simulink model "Model_turn"  (R2024a)
settings: Solver=VariableStepAuto  StartTime=0.0  StopTime=100  MaxStep=0.1  RelTol=1e-3
values from neighbouring files (symbols this model uses):
  c_SMA = 837.36    [params.m]
  Fmax_SMA = 10    [params.m]
  h_SMA = .3    (= 0.3)    [params.m]
  k_gn = m*g/0.01    (= 9810)    [contact3D_params.m]
  k_gt = m*g/0.1    (= 981)    [contact3D_params.m]
  m = 10    [contact3D_params.m]
  m_SMA = 0.0025    [params.m]
  max_SMA_Energy_J = 150    [params.m]
  mu_slide = 0.8    [contact3D_params.m]
  mu_stick = 0.9    [contact3D_params.m]
  n_segs = 10    [params.m]
  PWM_max = 0.35    [params.m]
  R_SMA = .08    (= 0.08)    [params.m]
  r_SMA2limb = 0.009    [params.m]
  swing_angle = swing_angles(i)    [params.m]
  T_amb = 23    [params.m]
  V_0 = 7    [params.m]
  v_gn_max = 0.03    [contact3D_params.m]
  v_gt_max = 0.03    [contact3D_params.m]
  vLimit = 0.01    [contact3D_params.m]
undefined symbols (not defined in the file or in its folder): Newton, Raphson, X, Y, Z
libraries: sm_lib x225, nesl_utility x185, simulink x24, simulink_extras x6
(part 2 of 16)

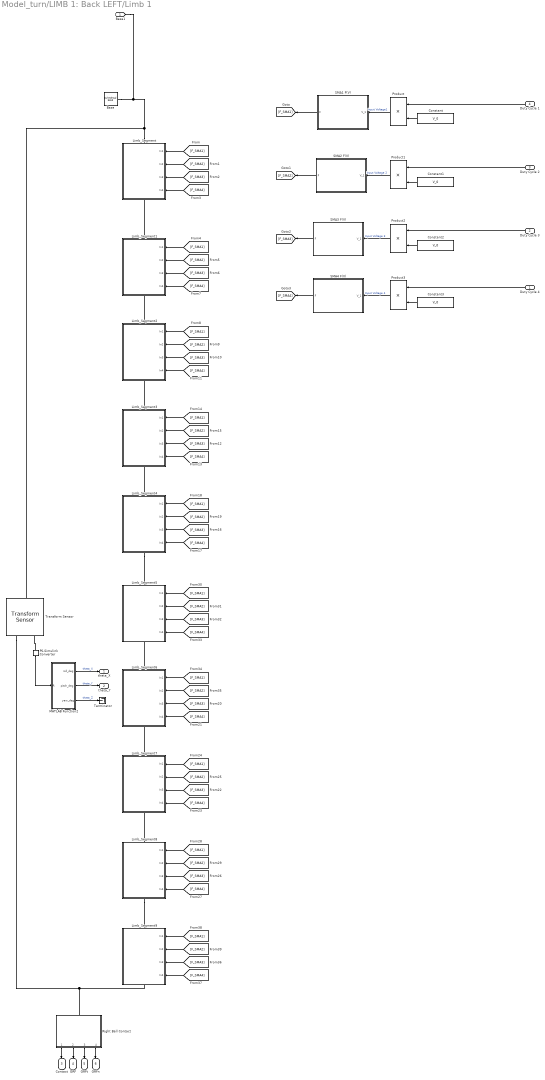
== system Model_turn/LIMB 1: Back LEFT/Limb 1 ==
  Duty Cycle 4 : Inport
  Duty Cycle 3 : Inport  Port=2
  Duty Cycle 2 : Inport  Port=3
  Duty Cycle 1 : Inport  Port=4
  Base : sm_lib/Body Elements/Cylindrical Solid  CylinderRadius=rad_limb  CylinderRadiusUnits=m  CylinderLength=seg_length  CylinderLengthUnits=m  ExportEntireGeometry=off  InertiaType=CalculateFromGeometry  BasedOnType=Density  Density=limb_density  DensityUnits=kg/m^3  Mass=1  MassUnits=kg  CenterOfMass=[0 0 0]  CenterOfMassUnits=m  MomentsOfInertia=[1 1 1]  MomentsOfInertiaUnits=kg*m^2  ProductsOfInertia=[0 0 0]  ProductsOfInertiaUnits=kg*m^2  GraphicType=FromGeometry  MarkerShape=Sphere  MarkerSize=10  GraphicVisPropType=SimpleVisualProperties  GraphicDiffuseColor=[0.5 0.5 0.5]  GraphicOpacity=1  GraphicSpecularColor=[0.5 0.5 0.5 1.0]  GraphicAmbientColor=[0.15 0.15 0.15 1.0]  GraphicEmissiveColor=[0.0 0.0 0.0 1.0]  GraphicShininess=75  DoExposeReferenceFrame=on  SerializedFrames=<Frames/>
  Constant{,1..3} (4 alike) : Constant  Value=V_0
  Limb_Segment : Subsystem
      settings: PortSchema="{\"entries\":[{\"content\":{\"sides\":[{\"content\":{\"connectorIds\":[\"In1\",\"In2\",\"In3\",\"In4\"]},\"type\":\"ConnectorPlacement.EquallySpacedRectSide\",\"uuid\":\"d6f10fa6-a397-4eb1-90c1-ee7478ada294\"},{\"content\":{\"side\":\"RIGHT\"},\"type\":\"ConnectorPlacement.EquallySpacedRectSide\",\"uuid\":\"3f1db35a-8e6d-4ba3-9e2d-f9910440e53b\"},{\"content\":{\"connectorIds\":[\"LConn1\"],\"side\":\"TOP\"},\"type\":\"ConnectorPlacement.EquallySpacedRectSide\",\"uuid\":\"a4104d1f-7883-4f84-b664-87694b536b33\"},{\"content\":{\"connectorIds\":[\"RConn1\"],\"side\":\"BOTTOM\"},\"type\":\"ConnectorPlacement.EquallySpacedRectSide\",\"uuid\":\"6469b369-5782-4c2c-b5b8-85624622bc1d\"}]},\"type\":\"ConnectorPlacement.EquallySpacedConnector\",\"uuid\":\"3cfa1fa9-4e06-4e7e-9a4a-6c954422b5b2\"}],\"packageUris\":[\"http://schema.mathworks.com/mf0/Connector/R2020b\"],\"version\":\"1.0\"}"
  Limb_Segment1 : Subsystem
      settings: PortSchema="{\"entries\":[{\"content\":{\"sides\":[{\"content\":{\"connectorIds\":[\"In1\",\"In2\",\"In3\",\"In4\"]},\"type\":\"ConnectorPlacement.EquallySpacedRectSide\",\"uuid\":\"d6f10fa6-a397-4eb1-90c1-ee7478ada294\"},{\"content\":{\"side\":\"RIGHT\"},\"type\":\"ConnectorPlacement.EquallySpacedRectSide\",\"uuid\":\"3f1db35a-8e6d-4ba3-9e2d-f9910440e53b\"},{\"content\":{\"connectorIds\":[\"LConn1\"],\"side\":\"TOP\"},\"type\":\"ConnectorPlacement.EquallySpacedRectSide\",\"uuid\":\"a4104d1f-7883-4f84-b664-87694b536b33\"},{\"content\":{\"connectorIds\":[\"RConn1\"],\"side\":\"BOTTOM\"},\"type\":\"ConnectorPlacement.EquallySpacedRectSide\",\"uuid\":\"6469b369-5782-4c2c-b5b8-85624622bc1d\"}]},\"type\":\"ConnectorPlacement.EquallySpacedConnector\",\"uuid\":\"3cfa1fa9-4e06-4e7e-9a4a-6c954422b5b2\"}],\"packageUris\":[\"http://schema.mathworks.com/mf0/Connector/R2020b\"],\"version\":\"1.0\"}"
  Limb_Segment2 : Subsystem
      settings: PortSchema="{\"entries\":[{\"content\":{\"sides\":[{\"content\":{\"connectorIds\":[\"In1\",\"In2\",\"In3\",\"In4\"]},\"type\":\"ConnectorPlacement.EquallySpacedRectSide\",\"uuid\":\"d6f10fa6-a397-4eb1-90c1-ee7478ada294\"},{\"content\":{\"side\":\"RIGHT\"},\"type\":\"ConnectorPlacement.EquallySpacedRectSide\",\"uuid\":\"3f1db35a-8e6d-4ba3-9e2d-f9910440e53b\"},{\"content\":{\"connectorIds\":[\"LConn1\"],\"side\":\"TOP\"},\"type\":\"ConnectorPlacement.EquallySpacedRectSide\",\"uuid\":\"a4104d1f-7883-4f84-b664-87694b536b33\"},{\"content\":{\"connectorIds\":[\"RConn1\"],\"side\":\"BOTTOM\"},\"type\":\"ConnectorPlacement.EquallySpacedRectSide\",\"uuid\":\"6469b369-5782-4c2c-b5b8-85624622bc1d\"}]},\"type\":\"ConnectorPlacement.EquallySpacedConnector\",\"uuid\":\"3cfa1fa9-4e06-4e7e-9a4a-6c954422b5b2\"}],\"packageUris\":[\"http://schema.mathworks.com/mf0/Connector/R2020b\"],\"version\":\"1.0\"}"
  Limb_Segment3 : Subsystem
      settings: PortSchema="{\"entries\":[{\"content\":{\"sides\":[{\"content\":{\"connectorIds\":[\"In1\",\"In2\",\"In3\",\"In4\"]},\"type\":\"ConnectorPlacement.EquallySpacedRectSide\",\"uuid\":\"d6f10fa6-a397-4eb1-90c1-ee7478ada294\"},{\"content\":{\"side\":\"RIGHT\"},\"type\":\"ConnectorPlacement.EquallySpacedRectSide\",\"uuid\":\"3f1db35a-8e6d-4ba3-9e2d-f9910440e53b\"},{\"content\":{\"connectorIds\":[\"LConn1\"],\"side\":\"TOP\"},\"type\":\"ConnectorPlacement.EquallySpacedRectSide\",\"uuid\":\"a4104d1f-7883-4f84-b664-87694b536b33\"},{\"content\":{\"connectorIds\":[\"RConn1\"],\"side\":\"BOTTOM\"},\"type\":\"ConnectorPlacement.EquallySpacedRectSide\",\"uuid\":\"6469b369-5782-4c2c-b5b8-85624622bc1d\"}]},\"type\":\"ConnectorPlacement.EquallySpacedConnector\",\"uuid\":\"3cfa1fa9-4e06-4e7e-9a4a-6c954422b5b2\"}],\"packageUris\":[\"http://schema.mathworks.com/mf0/Connector/R2020b\"],\"version\":\"1.0\"}"
  Limb_Segment4 : Subsystem
      settings: PortSchema="{\"entries\":[{\"content\":{\"sides\":[{\"content\":{\"connectorIds\":[\"In1\",\"In2\",\"In3\",\"In4\"]},\"type\":\"ConnectorPlacement.EquallySpacedRectSide\",\"uuid\":\"d6f10fa6-a397-4eb1-90c1-ee7478ada294\"},{\"content\":{\"side\":\"RIGHT\"},\"type\":\"ConnectorPlacement.EquallySpacedRectSide\",\"uuid\":\"3f1db35a-8e6d-4ba3-9e2d-f9910440e53b\"},{\"content\":{\"connectorIds\":[\"LConn1\"],\"side\":\"TOP\"},\"type\":\"ConnectorPlacement.EquallySpacedRectSide\",\"uuid\":\"a4104d1f-7883-4f84-b664-87694b536b33\"},{\"content\":{\"connectorIds\":[\"RConn1\"],\"side\":\"BOTTOM\"},\"type\":\"ConnectorPlacement.EquallySpacedRectSide\",\"uuid\":\"6469b369-5782-4c2c-b5b8-85624622bc1d\"}]},\"type\":\"ConnectorPlacement.EquallySpacedConnector\",\"uuid\":\"3cfa1fa9-4e06-4e7e-9a4a-6c954422b5b2\"}],\"packageUris\":[\"http://schema.mathworks.com/mf0/Connector/R2020b\"],\"version\":\"1.0\"}"
  Limb_Segment5 : Subsystem
      settings: PortSchema="{\"entries\":[{\"content\":{\"sides\":[{\"content\":{\"connectorIds\":[\"In1\",\"In2\",\"In3\",\"In4\"]},\"type\":\"ConnectorPlacement.EquallySpacedRectSide\",\"uuid\":\"d6f10fa6-a397-4eb1-90c1-ee7478ada294\"},{\"content\":{\"side\":\"RIGHT\"},\"type\":\"ConnectorPlacement.EquallySpacedRectSide\",\"uuid\":\"3f1db35a-8e6d-4ba3-9e2d-f9910440e53b\"},{\"content\":{\"connectorIds\":[\"LConn1\"],\"side\":\"TOP\"},\"type\":\"ConnectorPlacement.EquallySpacedRectSide\",\"uuid\":\"a4104d1f-7883-4f84-b664-87694b536b33\"},{\"content\":{\"connectorIds\":[\"RConn1\"],\"side\":\"BOTTOM\"},\"type\":\"ConnectorPlacement.EquallySpacedRectSide\",\"uuid\":\"6469b369-5782-4c2c-b5b8-85624622bc1d\"}]},\"type\":\"ConnectorPlacement.EquallySpacedConnector\",\"uuid\":\"3cfa1fa9-4e06-4e7e-9a4a-6c954422b5b2\"}],\"packageUris\":[\"http://schema.mathworks.com/mf0/Connector/R2020b\"],\"version\":\"1.0\"}"
  Limb_Segment6 : Subsystem
      settings: PortSchema="{\"entries\":[{\"content\":{\"sides\":[{\"content\":{\"connectorIds\":[\"In1\",\"In2\",\"In3\",\"In4\"]},\"type\":\"ConnectorPlacement.EquallySpacedRectSide\",\"uuid\":\"d6f10fa6-a397-4eb1-90c1-ee7478ada294\"},{\"content\":{\"side\":\"RIGHT\"},\"type\":\"ConnectorPlacement.EquallySpacedRectSide\",\"uuid\":\"3f1db35a-8e6d-4ba3-9e2d-f9910440e53b\"},{\"content\":{\"connectorIds\":[\"LConn1\"],\"side\":\"TOP\"},\"type\":\"ConnectorPlacement.EquallySpacedRectSide\",\"uuid\":\"a4104d1f-7883-4f84-b664-87694b536b33\"},{\"content\":{\"connectorIds\":[\"RConn1\"],\"side\":\"BOTTOM\"},\"type\":\"ConnectorPlacement.EquallySpacedRectSide\",\"uuid\":\"6469b369-5782-4c2c-b5b8-85624622bc1d\"}]},\"type\":\"ConnectorPlacement.EquallySpacedConnector\",\"uuid\":\"3cfa1fa9-4e06-4e7e-9a4a-6c954422b5b2\"}],\"packageUris\":[\"http://schema.mathworks.com/mf0/Connector/R2020b\"],\"version\":\"1.0\"}"
  Limb_Segment7 : Subsystem
      settings: PortSchema="{\"entries\":[{\"content\":{\"sides\":[{\"content\":{\"connectorIds\":[\"In1\",\"In2\",\"In3\",\"In4\"]},\"type\":\"ConnectorPlacement.EquallySpacedRectSide\",\"uuid\":\"d6f10fa6-a397-4eb1-90c1-ee7478ada294\"},{\"content\":{\"side\":\"RIGHT\"},\"type\":\"ConnectorPlacement.EquallySpacedRectSide\",\"uuid\":\"3f1db35a-8e6d-4ba3-9e2d-f9910440e53b\"},{\"content\":{\"connectorIds\":[\"LConn1\"],\"side\":\"TOP\"},\"type\":\"ConnectorPlacement.EquallySpacedRectSide\",\"uuid\":\"a4104d1f-7883-4f84-b664-87694b536b33\"},{\"content\":{\"connectorIds\":[\"RConn1\"],\"side\":\"BOTTOM\"},\"type\":\"ConnectorPlacement.EquallySpacedRectSide\",\"uuid\":\"6469b369-5782-4c2c-b5b8-85624622bc1d\"}]},\"type\":\"ConnectorPlacement.EquallySpacedConnector\",\"uuid\":\"3cfa1fa9-4e06-4e7e-9a4a-6c954422b5b2\"}],\"packageUris\":[\"http://schema.mathworks.com/mf0/Connector/R2020b\"],\"version\":\"1.0\"}"
  Limb_Segment8 : Subsystem
      settings: PortSchema="{\"entries\":[{\"content\":{\"sides\":[{\"content\":{\"connectorIds\":[\"In1\",\"In2\",\"In3\",\"In4\"]},\"type\":\"ConnectorPlacement.EquallySpacedRectSide\",\"uuid\":\"d6f10fa6-a397-4eb1-90c1-ee7478ada294\"},{\"content\":{\"side\":\"RIGHT\"},\"type\":\"ConnectorPlacement.EquallySpacedRectSide\",\"uuid\":\"3f1db35a-8e6d-4ba3-9e2d-f9910440e53b\"},{\"content\":{\"connectorIds\":[\"LConn1\"],\"side\":\"TOP\"},\"type\":\"ConnectorPlacement.EquallySpacedRectSide\",\"uuid\":\"a4104d1f-7883-4f84-b664-87694b536b33\"},{\"content\":{\"connectorIds\":[\"RConn1\"],\"side\":\"BOTTOM\"},\"type\":\"ConnectorPlacement.EquallySpacedRectSide\",\"uuid\":\"6469b369-5782-4c2c-b5b8-85624622bc1d\"}]},\"type\":\"ConnectorPlacement.EquallySpacedConnector\",\"uuid\":\"3cfa1fa9-4e06-4e7e-9a4a-6c954422b5b2\"}],\"packageUris\":[\"http://schema.mathworks.com/mf0/Connector/R2020b\"],\"version\":\"1.0\"}"
  Limb_Segment9 : Subsystem
      settings: PortSchema="{\"entries\":[{\"content\":{\"sides\":[{\"content\":{\"connectorIds\":[\"In1\",\"In2\",\"In3\",\"In4\"]},\"type\":\"ConnectorPlacement.EquallySpacedRectSide\",\"uuid\":\"d6f10fa6-a397-4eb1-90c1-ee7478ada294\"},{\"content\":{\"side\":\"RIGHT\"},\"type\":\"ConnectorPlacement.EquallySpacedRectSide\",\"uuid\":\"3f1db35a-8e6d-4ba3-9e2d-f9910440e53b\"},{\"content\":{\"connectorIds\":[\"LConn1\"],\"side\":\"TOP\"},\"type\":\"ConnectorPlacement.EquallySpacedRectSide\",\"uuid\":\"a4104d1f-7883-4f84-b664-87694b536b33\"},{\"content\":{\"connectorIds\":[\"RConn1\"],\"side\":\"BOTTOM\"},\"type\":\"ConnectorPlacement.EquallySpacedRectSide\",\"uuid\":\"6469b369-5782-4c2c-b5b8-85624622bc1d\"}]},\"type\":\"ConnectorPlacement.EquallySpacedConnector\",\"uuid\":\"3cfa1fa9-4e06-4e7e-9a4a-6c954422b5b2\"}],\"packageUris\":[\"http://schema.mathworks.com/mf0/Connector/R2020b\"],\"version\":\"1.0\"}"
  MATLAB Function2 : MATLAB Function  TreatAsAtomicUnit=on
  PS-Simulink Converter : nesl_utility/PS-Simulink Converter  PhysicalDomain=network_engine_domain  SubClassName=ps_output  LeftPortType=input  RightPortType=output  PseudoPeriodic=off  Frequencies=[]  VectorFormat=inherit  Unit=inherit  AffineConversion=off
  Product{,1..3} (4 alike) : Product
  Right Ball Contact : Subsystem
  SMA1 F(V) : Subsystem
  SMA2 F(V) : Subsystem
  SMA3 F(V) : Subsystem
  SMA4 F(V) : Subsystem
  Terminator : Terminator
  Transform Sensor : sm_lib/Frames and Transforms/Transform Sensor  MeasurementFrame=Base  RotationSequence=XYZ  SenseAngle=off  SenseAxis=off  SenseQ=off  SenseR=on  SenseRotationSequence=off  SenseOmegaX=off  SenseOmegaY=off  SenseOmegaZ=off  SenseOmega=off  SenseQDot=off  SenseRDot=off  SenseRotationSequenceDot=off  SenseAlphaX=off  SenseAlphaY=off  SenseAlphaZ=off  SenseAlpha=off  SenseQDDot=off  SenseRDDot=off  SenseX=off  SenseY=off  SenseZ=off  SenseXYZ=off  SenseRad=off  SenseAzim=off  SenseDist=off  SenseInc=off  SenseXDot=off  SenseYDot=off  SenseZDot=off  SenseXYZDot=off  SenseRadDot=off  SenseAzimDot=off  SenseDistDot=off  SenseIncDot=off  SenseXDDot=off  SenseYDDot=off  SenseZDDot=off  SenseXYZDDot=off  SenseRadDDot=off  SenseAzimDDot=off  SenseDistDDot=off  SenseIncDDot=off
  Base1 : PMIOPort  Side=Left
  theta_X : Outport
  theta_Y : Outport  Port=2
  "Contact " : Outport  Port=3
  GRF : Outport  Port=4
  GRFt : Outport  Port=5
  GRFn : Outport  Port=6
  wires:
  Duty Cycle 1/1 -> Product/1
  MATLAB Function2/1(roll_deg) -> theta_X/1  "theta_X"
  MATLAB Function2/2(pitch_deg) -> theta_Y/1  "theta_Y"
  Duty Cycle 2/1 -> Product1/1
  Duty Cycle 3/1 -> Product2/1
  Product1/1 -> SMA2 F(V)/1(V_1)  "Input Voltage 2"
  MATLAB Function2/3(yaw_deg) -> Terminator/1  "theta_Z"
  Product/1 -> SMA1 F(V)/1(V_1)  "Input Voltage1"
  Constant3/1 -> Product3/2
  [F_SMA2] -> Limb_Segment5/2(In2)
  [F_SMA4] -> Limb_Segment7/4(In4)
  [F_SMA4] -> Limb_Segment/4(In4)
  [F_SMA4] -> Limb_Segment2/4(In4)
  [F_SMA1] -> Limb_Segment7/1(In1)
  [F_SMA3] -> Limb_Segment6/3(In3)
  SMA4 F(V)/1(F) -> [F_SMA4]
  [F_SMA1] -> Limb_Segment9/1(In1)
  [F_SMA4] -> Limb_Segment9/4(In4)
  Constant1/1 -> Product1/2
  [F_SMA3] -> Limb_Segment3/3(In3)
  [F_SMA2] -> Limb_Segment6/2(In2)
  Product3/1 -> SMA4 F(V)/1(V_1)  "Input Voltage 4"
  [F_SMA1] -> Limb_Segment/1(In1)
  PS-Simulink Converter/1 -> MATLAB Function2/1(R)
  [F_SMA4] -> Limb_Segment6/4(In4)
  [F_SMA3] -> Limb_Segment8/3(In3)
  [F_SMA1] -> Limb_Segment8/1(In1)
  [F_SMA1] -> Limb_Segment3/1(In1)
  Duty Cycle 4/1 -> Product3/1
  [F_SMA1] -> Limb_Segment5/1(In1)
  [F_SMA1] -> Limb_Segment4/1(In1)
  [F_SMA2] -> Limb_Segment7/2(In2)
  [F_SMA2] -> Limb_Segment2/2(In2)
  SMA2 F(V)/1(F) -> [F_SMA2]
  Product2/1 -> SMA3 F(V)/1(V_1)  "Input Voltage 3"
  [F_SMA3] -> Limb_Segment9/3(In3)
  [F_SMA2] -> Limb_Segment1/2(In2)
  [F_SMA1] -> Limb_Segment2/1(In1)
  [F_SMA3] -> Limb_Segment4/3(In3)
  [F_SMA2] -> Limb_Segment/2(In2)
  [F_SMA3] -> Limb_Segment/3(In3)
  [F_SMA4] -> Limb_Segment3/4(In4)
  [F_SMA4] -> Limb_Segment1/4(In4)
  [F_SMA4] -> Limb_Segment5/4(In4)
  [F_SMA4] -> Limb_Segment4/4(In4)
  Constant/1 -> Product/2
  [F_SMA3] -> Limb_Segment7/3(In3)
  [F_SMA3] -> Limb_Segment5/3(In3)
  [F_SMA4] -> Limb_Segment8/4(In4)
  SMA1 F(V)/1(F) -> [F_SMA1]
  [F_SMA1] -> Limb_Segment6/1(In1)
  Constant2/1 -> Product2/2
  [F_SMA2] -> Limb_Segment9/2(In2)
  [F_SMA3] -> Limb_Segment1/3(In3)
  SMA3 F(V)/1(F) -> [F_SMA3]
  [F_SMA3] -> Limb_Segment2/3(In3)
  [F_SMA2] -> Limb_Segment8/2(In2)
  [F_SMA1] -> Limb_Segment1/1(In1)
  [F_SMA2] -> Limb_Segment3/2(In2)
  [F_SMA2] -> Limb_Segment4/2(In2)
  Right Ball Contact/2(GRF [N N N]) -> GRF/1
  Right Ball Contact/4(GRFn [N N N]) -> GRFn/1
  Right Ball Contact/1(RBallContact [bool]) -> "Contact "/1
  Right Ball Contact/3(GRFt [N N N]) -> GRFt/1
  connections:
  PS-Simulink Converter/LConn1 -- Transform Sensor/RConn2
  Limb_Segment1/LConn1 -- Limb_Segment/RConn1
  Limb_Segment4/RConn1 -- Limb_Segment5/LConn1
  Limb_Segment7/LConn1 -- Limb_Segment6/RConn1
  Transform Sensor/RConn1 -- Right Ball Contact/LConn1 -- Limb_Segment9/RConn1
  Limb_Segment8/LConn1 -- Limb_Segment7/RConn1
  Limb_Segment6/LConn1 -- Limb_Segment5/RConn1
  Limb_Segment4/LConn1 -- Limb_Segment3/RConn1
  Limb_Segment3/LConn1 -- Limb_Segment2/RConn1
  Limb_Segment8/RConn1 -- Limb_Segment9/LConn1
  Limb_Segment2/LConn1 -- Limb_Segment1/RConn1
  Limb_Segment/LConn1 -- Base/RConn1 -- Base1/RConn1 -- Transform Sensor/LConn1

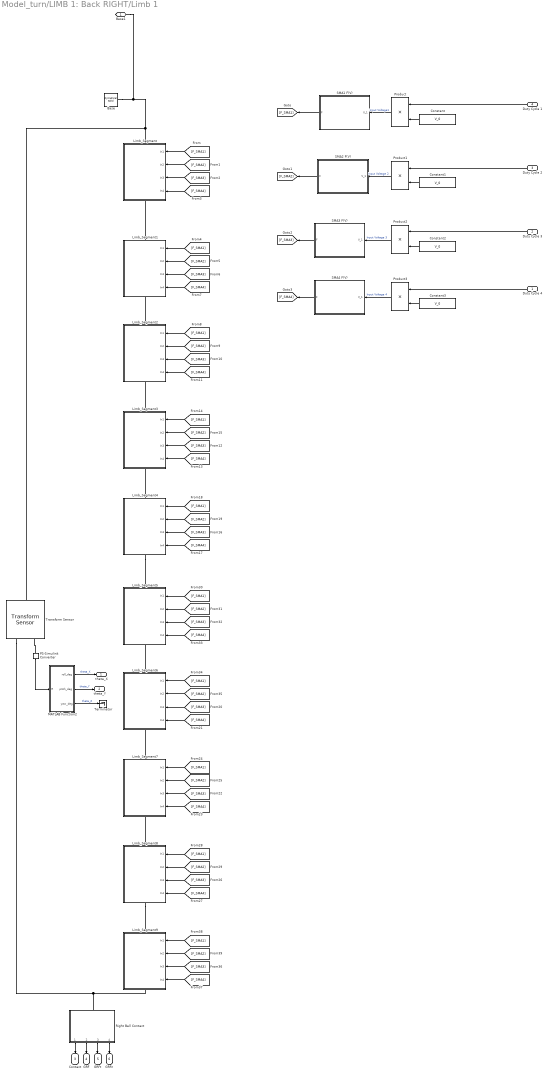
== system Model_turn/LIMB 1: Back RIGHT/Limb 1 ==
  Duty Cycle 4 : Inport
  Duty Cycle 3 : Inport  Port=2
  Duty Cycle 2 : Inport  Port=3
  Duty Cycle 1 : Inport  Port=4
  Base : sm_lib/Body Elements/Cylindrical Solid  CylinderRadius=rad_limb  CylinderRadiusUnits=m  CylinderLength=seg_length  CylinderLengthUnits=m  ExportEntireGeometry=off  InertiaType=CalculateFromGeometry  BasedOnType=Density  Density=limb_density  DensityUnits=kg/m^3  Mass=1  MassUnits=kg  CenterOfMass=[0 0 0]  CenterOfMassUnits=m  MomentsOfInertia=[1 1 1]  MomentsOfInertiaUnits=kg*m^2  ProductsOfInertia=[0 0 0]  ProductsOfInertiaUnits=kg*m^2  GraphicType=FromGeometry  MarkerShape=Sphere  MarkerSize=10  GraphicVisPropType=SimpleVisualProperties  GraphicDiffuseColor=[0.5 0.5 0.5]  GraphicOpacity=1  GraphicSpecularColor=[0.5 0.5 0.5 1.0]  GraphicAmbientColor=[0.15 0.15 0.15 1.0]  GraphicEmissiveColor=[0.0 0.0 0.0 1.0]  GraphicShininess=75  DoExposeReferenceFrame=on  SerializedFrames=<Frames/>
  Constant{,1..3} (4 alike) : Constant  Value=V_0
  Limb_Segment : Subsystem
      settings: PortSchema="{\"entries\":[{\"content\":{\"sides\":[{\"content\":{\"connectorIds\":[\"In1\",\"In2\",\"In3\",\"In4\"]},\"type\":\"ConnectorPlacement.EquallySpacedRectSide\",\"uuid\":\"d6f10fa6-a397-4eb1-90c1-ee7478ada294\"},{\"content\":{\"side\":\"RIGHT\"},\"type\":\"ConnectorPlacement.EquallySpacedRectSide\",\"uuid\":\"3f1db35a-8e6d-4ba3-9e2d-f9910440e53b\"},{\"content\":{\"connectorIds\":[\"LConn1\"],\"side\":\"TOP\"},\"type\":\"ConnectorPlacement.EquallySpacedRectSide\",\"uuid\":\"a4104d1f-7883-4f84-b664-87694b536b33\"},{\"content\":{\"connectorIds\":[\"RConn1\"],\"side\":\"BOTTOM\"},\"type\":\"ConnectorPlacement.EquallySpacedRectSide\",\"uuid\":\"6469b369-5782-4c2c-b5b8-85624622bc1d\"}]},\"type\":\"ConnectorPlacement.EquallySpacedConnector\",\"uuid\":\"3cfa1fa9-4e06-4e7e-9a4a-6c954422b5b2\"}],\"packageUris\":[\"http://schema.mathworks.com/mf0/Connector/R2020b\"],\"version\":\"1.0\"}"
  Limb_Segment1 : Subsystem
      settings: PortSchema="{\"entries\":[{\"content\":{\"sides\":[{\"content\":{\"connectorIds\":[\"In1\",\"In2\",\"In3\",\"In4\"]},\"type\":\"ConnectorPlacement.EquallySpacedRectSide\",\"uuid\":\"d6f10fa6-a397-4eb1-90c1-ee7478ada294\"},{\"content\":{\"side\":\"RIGHT\"},\"type\":\"ConnectorPlacement.EquallySpacedRectSide\",\"uuid\":\"3f1db35a-8e6d-4ba3-9e2d-f9910440e53b\"},{\"content\":{\"connectorIds\":[\"LConn1\"],\"side\":\"TOP\"},\"type\":\"ConnectorPlacement.EquallySpacedRectSide\",\"uuid\":\"a4104d1f-7883-4f84-b664-87694b536b33\"},{\"content\":{\"connectorIds\":[\"RConn1\"],\"side\":\"BOTTOM\"},\"type\":\"ConnectorPlacement.EquallySpacedRectSide\",\"uuid\":\"6469b369-5782-4c2c-b5b8-85624622bc1d\"}]},\"type\":\"ConnectorPlacement.EquallySpacedConnector\",\"uuid\":\"3cfa1fa9-4e06-4e7e-9a4a-6c954422b5b2\"}],\"packageUris\":[\"http://schema.mathworks.com/mf0/Connector/R2020b\"],\"version\":\"1.0\"}"
  Limb_Segment2 : Subsystem
      settings: PortSchema="{\"entries\":[{\"content\":{\"sides\":[{\"content\":{\"connectorIds\":[\"In1\",\"In2\",\"In3\",\"In4\"]},\"type\":\"ConnectorPlacement.EquallySpacedRectSide\",\"uuid\":\"d6f10fa6-a397-4eb1-90c1-ee7478ada294\"},{\"content\":{\"side\":\"RIGHT\"},\"type\":\"ConnectorPlacement.EquallySpacedRectSide\",\"uuid\":\"3f1db35a-8e6d-4ba3-9e2d-f9910440e53b\"},{\"content\":{\"connectorIds\":[\"LConn1\"],\"side\":\"TOP\"},\"type\":\"ConnectorPlacement.EquallySpacedRectSide\",\"uuid\":\"a4104d1f-7883-4f84-b664-87694b536b33\"},{\"content\":{\"connectorIds\":[\"RConn1\"],\"side\":\"BOTTOM\"},\"type\":\"ConnectorPlacement.EquallySpacedRectSide\",\"uuid\":\"6469b369-5782-4c2c-b5b8-85624622bc1d\"}]},\"type\":\"ConnectorPlacement.EquallySpacedConnector\",\"uuid\":\"3cfa1fa9-4e06-4e7e-9a4a-6c954422b5b2\"}],\"packageUris\":[\"http://schema.mathworks.com/mf0/Connector/R2020b\"],\"version\":\"1.0\"}"
  Limb_Segment3 : Subsystem
      settings: PortSchema="{\"entries\":[{\"content\":{\"sides\":[{\"content\":{\"connectorIds\":[\"In1\",\"In2\",\"In3\",\"In4\"]},\"type\":\"ConnectorPlacement.EquallySpacedRectSide\",\"uuid\":\"d6f10fa6-a397-4eb1-90c1-ee7478ada294\"},{\"content\":{\"side\":\"RIGHT\"},\"type\":\"ConnectorPlacement.EquallySpacedRectSide\",\"uuid\":\"3f1db35a-8e6d-4ba3-9e2d-f9910440e53b\"},{\"content\":{\"connectorIds\":[\"LConn1\"],\"side\":\"TOP\"},\"type\":\"ConnectorPlacement.EquallySpacedRectSide\",\"uuid\":\"a4104d1f-7883-4f84-b664-87694b536b33\"},{\"content\":{\"connectorIds\":[\"RConn1\"],\"side\":\"BOTTOM\"},\"type\":\"ConnectorPlacement.EquallySpacedRectSide\",\"uuid\":\"6469b369-5782-4c2c-b5b8-85624622bc1d\"}]},\"type\":\"ConnectorPlacement.EquallySpacedConnector\",\"uuid\":\"3cfa1fa9-4e06-4e7e-9a4a-6c954422b5b2\"}],\"packageUris\":[\"http://schema.mathworks.com/mf0/Connector/R2020b\"],\"version\":\"1.0\"}"
  Limb_Segment4 : Subsystem
      settings: PortSchema="{\"entries\":[{\"content\":{\"sides\":[{\"content\":{\"connectorIds\":[\"In1\",\"In2\",\"In3\",\"In4\"]},\"type\":\"ConnectorPlacement.EquallySpacedRectSide\",\"uuid\":\"d6f10fa6-a397-4eb1-90c1-ee7478ada294\"},{\"content\":{\"side\":\"RIGHT\"},\"type\":\"ConnectorPlacement.EquallySpacedRectSide\",\"uuid\":\"3f1db35a-8e6d-4ba3-9e2d-f9910440e53b\"},{\"content\":{\"connectorIds\":[\"LConn1\"],\"side\":\"TOP\"},\"type\":\"ConnectorPlacement.EquallySpacedRectSide\",\"uuid\":\"a4104d1f-7883-4f84-b664-87694b536b33\"},{\"content\":{\"connectorIds\":[\"RConn1\"],\"side\":\"BOTTOM\"},\"type\":\"ConnectorPlacement.EquallySpacedRectSide\",\"uuid\":\"6469b369-5782-4c2c-b5b8-85624622bc1d\"}]},\"type\":\"ConnectorPlacement.EquallySpacedConnector\",\"uuid\":\"3cfa1fa9-4e06-4e7e-9a4a-6c954422b5b2\"}],\"packageUris\":[\"http://schema.mathworks.com/mf0/Connector/R2020b\"],\"version\":\"1.0\"}"
  Limb_Segment5 : Subsystem
      settings: PortSchema="{\"entries\":[{\"content\":{\"sides\":[{\"content\":{\"connectorIds\":[\"In1\",\"In2\",\"In3\",\"In4\"]},\"type\":\"ConnectorPlacement.EquallySpacedRectSide\",\"uuid\":\"d6f10fa6-a397-4eb1-90c1-ee7478ada294\"},{\"content\":{\"side\":\"RIGHT\"},\"type\":\"ConnectorPlacement.EquallySpacedRectSide\",\"uuid\":\"3f1db35a-8e6d-4ba3-9e2d-f9910440e53b\"},{\"content\":{\"connectorIds\":[\"LConn1\"],\"side\":\"TOP\"},\"type\":\"ConnectorPlacement.EquallySpacedRectSide\",\"uuid\":\"a4104d1f-7883-4f84-b664-87694b536b33\"},{\"content\":{\"connectorIds\":[\"RConn1\"],\"side\":\"BOTTOM\"},\"type\":\"ConnectorPlacement.EquallySpacedRectSide\",\"uuid\":\"6469b369-5782-4c2c-b5b8-85624622bc1d\"}]},\"type\":\"ConnectorPlacement.EquallySpacedConnector\",\"uuid\":\"3cfa1fa9-4e06-4e7e-9a4a-6c954422b5b2\"}],\"packageUris\":[\"http://schema.mathworks.com/mf0/Connector/R2020b\"],\"version\":\"1.0\"}"
  Limb_Segment6 : Subsystem
      settings: PortSchema="{\"entries\":[{\"content\":{\"sides\":[{\"content\":{\"connectorIds\":[\"In1\",\"In2\",\"In3\",\"In4\"]},\"type\":\"ConnectorPlacement.EquallySpacedRectSide\",\"uuid\":\"d6f10fa6-a397-4eb1-90c1-ee7478ada294\"},{\"content\":{\"side\":\"RIGHT\"},\"type\":\"ConnectorPlacement.EquallySpacedRectSide\",\"uuid\":\"3f1db35a-8e6d-4ba3-9e2d-f9910440e53b\"},{\"content\":{\"connectorIds\":[\"LConn1\"],\"side\":\"TOP\"},\"type\":\"ConnectorPlacement.EquallySpacedRectSide\",\"uuid\":\"a4104d1f-7883-4f84-b664-87694b536b33\"},{\"content\":{\"connectorIds\":[\"RConn1\"],\"side\":\"BOTTOM\"},\"type\":\"ConnectorPlacement.EquallySpacedRectSide\",\"uuid\":\"6469b369-5782-4c2c-b5b8-85624622bc1d\"}]},\"type\":\"ConnectorPlacement.EquallySpacedConnector\",\"uuid\":\"3cfa1fa9-4e06-4e7e-9a4a-6c954422b5b2\"}],\"packageUris\":[\"http://schema.mathworks.com/mf0/Connector/R2020b\"],\"version\":\"1.0\"}"
  Limb_Segment7 : Subsystem
      settings: PortSchema="{\"entries\":[{\"content\":{\"sides\":[{\"content\":{\"connectorIds\":[\"In1\",\"In2\",\"In3\",\"In4\"]},\"type\":\"ConnectorPlacement.EquallySpacedRectSide\",\"uuid\":\"d6f10fa6-a397-4eb1-90c1-ee7478ada294\"},{\"content\":{\"side\":\"RIGHT\"},\"type\":\"ConnectorPlacement.EquallySpacedRectSide\",\"uuid\":\"3f1db35a-8e6d-4ba3-9e2d-f9910440e53b\"},{\"content\":{\"connectorIds\":[\"LConn1\"],\"side\":\"TOP\"},\"type\":\"ConnectorPlacement.EquallySpacedRectSide\",\"uuid\":\"a4104d1f-7883-4f84-b664-87694b536b33\"},{\"content\":{\"connectorIds\":[\"RConn1\"],\"side\":\"BOTTOM\"},\"type\":\"ConnectorPlacement.EquallySpacedRectSide\",\"uuid\":\"6469b369-5782-4c2c-b5b8-85624622bc1d\"}]},\"type\":\"ConnectorPlacement.EquallySpacedConnector\",\"uuid\":\"3cfa1fa9-4e06-4e7e-9a4a-6c954422b5b2\"}],\"packageUris\":[\"http://schema.mathworks.com/mf0/Connector/R2020b\"],\"version\":\"1.0\"}"
  Limb_Segment8 : Subsystem
      settings: PortSchema="{\"entries\":[{\"content\":{\"sides\":[{\"content\":{\"connectorIds\":[\"In1\",\"In2\",\"In3\",\"In4\"]},\"type\":\"ConnectorPlacement.EquallySpacedRectSide\",\"uuid\":\"d6f10fa6-a397-4eb1-90c1-ee7478ada294\"},{\"content\":{\"side\":\"RIGHT\"},\"type\":\"ConnectorPlacement.EquallySpacedRectSide\",\"uuid\":\"3f1db35a-8e6d-4ba3-9e2d-f9910440e53b\"},{\"content\":{\"connectorIds\":[\"LConn1\"],\"side\":\"TOP\"},\"type\":\"ConnectorPlacement.EquallySpacedRectSide\",\"uuid\":\"a4104d1f-7883-4f84-b664-87694b536b33\"},{\"content\":{\"connectorIds\":[\"RConn1\"],\"side\":\"BOTTOM\"},\"type\":\"ConnectorPlacement.EquallySpacedRectSide\",\"uuid\":\"6469b369-5782-4c2c-b5b8-85624622bc1d\"}]},\"type\":\"ConnectorPlacement.EquallySpacedConnector\",\"uuid\":\"3cfa1fa9-4e06-4e7e-9a4a-6c954422b5b2\"}],\"packageUris\":[\"http://schema.mathworks.com/mf0/Connector/R2020b\"],\"version\":\"1.0\"}"
  Limb_Segment9 : Subsystem
      settings: PortSchema="{\"entries\":[{\"content\":{\"sides\":[{\"content\":{\"connectorIds\":[\"In1\",\"In2\",\"In3\",\"In4\"]},\"type\":\"ConnectorPlacement.EquallySpacedRectSide\",\"uuid\":\"d6f10fa6-a397-4eb1-90c1-ee7478ada294\"},{\"content\":{\"side\":\"RIGHT\"},\"type\":\"ConnectorPlacement.EquallySpacedRectSide\",\"uuid\":\"3f1db35a-8e6d-4ba3-9e2d-f9910440e53b\"},{\"content\":{\"connectorIds\":[\"LConn1\"],\"side\":\"TOP\"},\"type\":\"ConnectorPlacement.EquallySpacedRectSide\",\"uuid\":\"a4104d1f-7883-4f84-b664-87694b536b33\"},{\"content\":{\"connectorIds\":[\"RConn1\"],\"side\":\"BOTTOM\"},\"type\":\"ConnectorPlacement.EquallySpacedRectSide\",\"uuid\":\"6469b369-5782-4c2c-b5b8-85624622bc1d\"}]},\"type\":\"ConnectorPlacement.EquallySpacedConnector\",\"uuid\":\"3cfa1fa9-4e06-4e7e-9a4a-6c954422b5b2\"}],\"packageUris\":[\"http://schema.mathworks.com/mf0/Connector/R2020b\"],\"version\":\"1.0\"}"
  MATLAB Function2 : MATLAB Function  TreatAsAtomicUnit=on
  PS-Simulink Converter : nesl_utility/PS-Simulink Converter  PhysicalDomain=network_engine_domain  SubClassName=ps_output  LeftPortType=input  RightPortType=output  PseudoPeriodic=off  Frequencies=[]  VectorFormat=inherit  Unit=inherit  AffineConversion=off
  Product{,1..3} (4 alike) : Product
  Right Ball Contact : Subsystem
  SMA1 F(V) : Subsystem
  SMA2 F(V) : Subsystem
  SMA3 F(V) : Subsystem
  SMA4 F(V) : Subsystem
  Terminator : Terminator
  Transform Sensor : sm_lib/Frames and Transforms/Transform Sensor  MeasurementFrame=Base  RotationSequence=XYZ  SenseAngle=off  SenseAxis=off  SenseQ=off  SenseR=on  SenseRotationSequence=off  SenseOmegaX=off  SenseOmegaY=off  SenseOmegaZ=off  SenseOmega=off  SenseQDot=off  SenseRDot=off  SenseRotationSequenceDot=off  SenseAlphaX=off  SenseAlphaY=off  SenseAlphaZ=off  SenseAlpha=off  SenseQDDot=off  SenseRDDot=off  SenseX=off  SenseY=off  SenseZ=off  SenseXYZ=off  SenseRad=off  SenseAzim=off  SenseDist=off  SenseInc=off  SenseXDot=off  SenseYDot=off  SenseZDot=off  SenseXYZDot=off  SenseRadDot=off  SenseAzimDot=off  SenseDistDot=off  SenseIncDot=off  SenseXDDot=off  SenseYDDot=off  SenseZDDot=off  SenseXYZDDot=off  SenseRadDDot=off  SenseAzimDDot=off  SenseDistDDot=off  SenseIncDDot=off
  Base1 : PMIOPort  Side=Left
  theta_X : Outport
  theta_Y : Outport  Port=2
  "Contact " : Outport  Port=3
  GRF : Outport  Port=4
  GRFt : Outport  Port=5
  GRFn : Outport  Port=6
  wires:
  [F_SMA2] -> Limb_Segment4/2(In2)
  [F_SMA2] -> Limb_Segment3/2(In2)
  [F_SMA1] -> Limb_Segment1/1(In1)
  [F_SMA2] -> Limb_Segment8/2(In2)
  [F_SMA3] -> Limb_Segment2/3(In3)
  SMA3 F(V)/1(F) -> [F_SMA3]
  [F_SMA3] -> Limb_Segment1/3(In3)
  [F_SMA2] -> Limb_Segment9/2(In2)
  Constant2/1 -> Product2/2
  [F_SMA1] -> Limb_Segment6/1(In1)
  SMA1 F(V)/1(F) -> [F_SMA1]
  [F_SMA4] -> Limb_Segment8/4(In4)
  [F_SMA3] -> Limb_Segment5/3(In3)
  [F_SMA3] -> Limb_Segment7/3(In3)
  Constant/1 -> Product/2
  [F_SMA4] -> Limb_Segment4/4(In4)
  [F_SMA4] -> Limb_Segment5/4(In4)
  [F_SMA4] -> Limb_Segment1/4(In4)
  [F_SMA4] -> Limb_Segment3/4(In4)
  [F_SMA3] -> Limb_Segment/3(In3)
  [F_SMA2] -> Limb_Segment/2(In2)
  [F_SMA3] -> Limb_Segment4/3(In3)
  [F_SMA1] -> Limb_Segment2/1(In1)
  [F_SMA2] -> Limb_Segment1/2(In2)
  [F_SMA3] -> Limb_Segment9/3(In3)
  Product2/1 -> SMA3 F(V)/1(V_1)  "Input Voltage 3"
  SMA2 F(V)/1(F) -> [F_SMA2]
  [F_SMA2] -> Limb_Segment2/2(In2)
  [F_SMA2] -> Limb_Segment7/2(In2)
  [F_SMA1] -> Limb_Segment4/1(In1)
  [F_SMA1] -> Limb_Segment5/1(In1)
  Duty Cycle 4/1 -> Product3/1
  [F_SMA1] -> Limb_Segment3/1(In1)
  [F_SMA1] -> Limb_Segment8/1(In1)
  [F_SMA3] -> Limb_Segment8/3(In3)
  [F_SMA4] -> Limb_Segment6/4(In4)
  PS-Simulink Converter/1 -> MATLAB Function2/1(R)
  [F_SMA1] -> Limb_Segment/1(In1)
  Product3/1 -> SMA4 F(V)/1(V_1)  "Input Voltage 4"
  [F_SMA2] -> Limb_Segment6/2(In2)
  [F_SMA3] -> Limb_Segment3/3(In3)
  Constant1/1 -> Product1/2
  [F_SMA4] -> Limb_Segment9/4(In4)
  [F_SMA1] -> Limb_Segment9/1(In1)
  SMA4 F(V)/1(F) -> [F_SMA4]
  [F_SMA3] -> Limb_Segment6/3(In3)
  [F_SMA1] -> Limb_Segment7/1(In1)
  [F_SMA4] -> Limb_Segment2/4(In4)
  [F_SMA4] -> Limb_Segment/4(In4)
  [F_SMA4] -> Limb_Segment7/4(In4)
  [F_SMA2] -> Limb_Segment5/2(In2)
  Constant3/1 -> Product3/2
  Product/1 -> SMA1 F(V)/1(V_1)  "Input Voltage1"
  MATLAB Function2/3(yaw_deg) -> Terminator/1  "theta_Z"
  Product1/1 -> SMA2 F(V)/1(V_1)  "Input Voltage 2"
  Duty Cycle 3/1 -> Product2/1
  Duty Cycle 2/1 -> Product1/1
  MATLAB Function2/2(pitch_deg) -> theta_Y/1  "theta_Y"
  MATLAB Function2/1(roll_deg) -> theta_X/1  "theta_X"
  Duty Cycle 1/1 -> Product/1
  Right Ball Contact/2(GRF [N N N]) -> GRF/1
  Right Ball Contact/4(GRFn [N N N]) -> GRFn/1
  Right Ball Contact/1(RBallContact [bool]) -> "Contact "/1
  Right Ball Contact/3(GRFt [N N N]) -> GRFt/1
  connections:
  Transform Sensor/LConn1 -- Base1/RConn1 -- Base/RConn1 -- Limb_Segment/LConn1
  Limb_Segment2/LConn1 -- Limb_Segment1/RConn1
  Limb_Segment8/RConn1 -- Limb_Segment9/LConn1
  Limb_Segment3/LConn1 -- Limb_Segment2/RConn1
  Limb_Segment4/LConn1 -- Limb_Segment3/RConn1
  Limb_Segment6/LConn1 -- Limb_Segment5/RConn1
  Limb_Segment8/LConn1 -- Limb_Segment7/RConn1
  Transform Sensor/RConn1 -- Right Ball Contact/LConn1 -- Limb_Segment9/RConn1
  Limb_Segment7/LConn1 -- Limb_Segment6/RConn1
  Limb_Segment4/RConn1 -- Limb_Segment5/LConn1
  Limb_Segment1/LConn1 -- Limb_Segment/RConn1
  PS-Simulink Converter/LConn1 -- Transform Sensor/RConn2

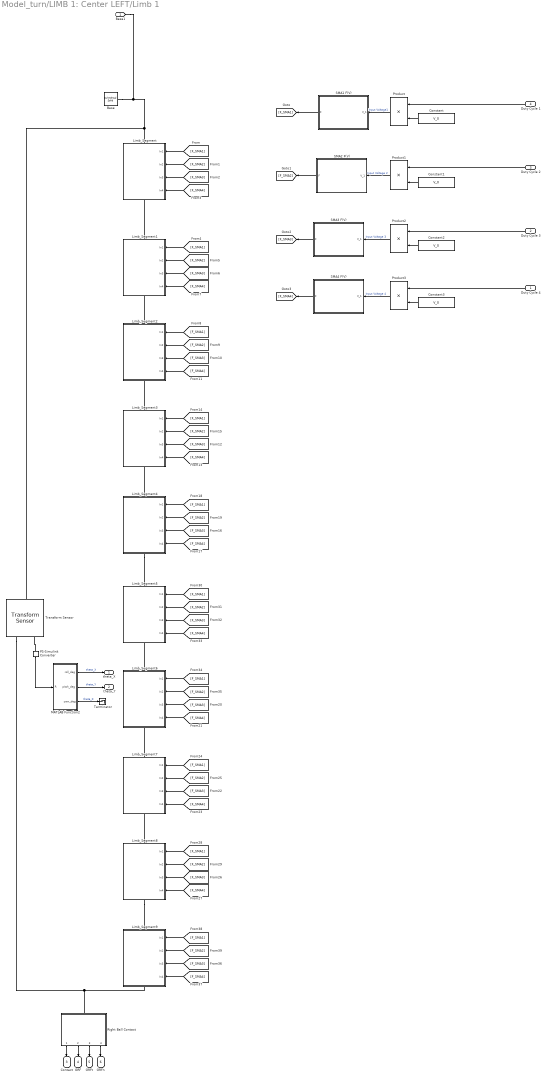
== system Model_turn/LIMB 1: Center LEFT/Limb 1 ==
  Duty Cycle 4 : Inport
  Duty Cycle 3 : Inport  Port=2
  Duty Cycle 2 : Inport  Port=3
  Duty Cycle 1 : Inport  Port=4
  Base : sm_lib/Body Elements/Cylindrical Solid  CylinderRadius=rad_limb  CylinderRadiusUnits=m  CylinderLength=seg_length  CylinderLengthUnits=m  ExportEntireGeometry=off  InertiaType=CalculateFromGeometry  BasedOnType=Density  Density=limb_density  DensityUnits=kg/m^3  Mass=1  MassUnits=kg  CenterOfMass=[0 0 0]  CenterOfMassUnits=m  MomentsOfInertia=[1 1 1]  MomentsOfInertiaUnits=kg*m^2  ProductsOfInertia=[0 0 0]  ProductsOfInertiaUnits=kg*m^2  GraphicType=FromGeometry  MarkerShape=Sphere  MarkerSize=10  GraphicVisPropType=SimpleVisualProperties  GraphicDiffuseColor=[0.5 0.5 0.5]  GraphicOpacity=1  GraphicSpecularColor=[0.5 0.5 0.5 1.0]  GraphicAmbientColor=[0.15 0.15 0.15 1.0]  GraphicEmissiveColor=[0.0 0.0 0.0 1.0]  GraphicShininess=75  DoExposeReferenceFrame=on  SerializedFrames=<Frames/>
  Constant{,1..3} (4 alike) : Constant  Value=V_0
  Limb_Segment : Subsystem
      settings: PortSchema="{\"entries\":[{\"content\":{\"sides\":[{\"content\":{\"connectorIds\":[\"In1\",\"In2\",\"In3\",\"In4\"]},\"type\":\"ConnectorPlacement.EquallySpacedRectSide\",\"uuid\":\"d6f10fa6-a397-4eb1-90c1-ee7478ada294\"},{\"content\":{\"side\":\"RIGHT\"},\"type\":\"ConnectorPlacement.EquallySpacedRectSide\",\"uuid\":\"3f1db35a-8e6d-4ba3-9e2d-f9910440e53b\"},{\"content\":{\"connectorIds\":[\"LConn1\"],\"side\":\"TOP\"},\"type\":\"ConnectorPlacement.EquallySpacedRectSide\",\"uuid\":\"a4104d1f-7883-4f84-b664-87694b536b33\"},{\"content\":{\"connectorIds\":[\"RConn1\"],\"side\":\"BOTTOM\"},\"type\":\"ConnectorPlacement.EquallySpacedRectSide\",\"uuid\":\"6469b369-5782-4c2c-b5b8-85624622bc1d\"}]},\"type\":\"ConnectorPlacement.EquallySpacedConnector\",\"uuid\":\"3cfa1fa9-4e06-4e7e-9a4a-6c954422b5b2\"}],\"packageUris\":[\"http://schema.mathworks.com/mf0/Connector/R2020b\"],\"version\":\"1.0\"}"
  Limb_Segment1 : Subsystem
      settings: PortSchema="{\"entries\":[{\"content\":{\"sides\":[{\"content\":{\"connectorIds\":[\"In1\",\"In2\",\"In3\",\"In4\"]},\"type\":\"ConnectorPlacement.EquallySpacedRectSide\",\"uuid\":\"d6f10fa6-a397-4eb1-90c1-ee7478ada294\"},{\"content\":{\"side\":\"RIGHT\"},\"type\":\"ConnectorPlacement.EquallySpacedRectSide\",\"uuid\":\"3f1db35a-8e6d-4ba3-9e2d-f9910440e53b\"},{\"content\":{\"connectorIds\":[\"LConn1\"],\"side\":\"TOP\"},\"type\":\"ConnectorPlacement.EquallySpacedRectSide\",\"uuid\":\"a4104d1f-7883-4f84-b664-87694b536b33\"},{\"content\":{\"connectorIds\":[\"RConn1\"],\"side\":\"BOTTOM\"},\"type\":\"ConnectorPlacement.EquallySpacedRectSide\",\"uuid\":\"6469b369-5782-4c2c-b5b8-85624622bc1d\"}]},\"type\":\"ConnectorPlacement.EquallySpacedConnector\",\"uuid\":\"3cfa1fa9-4e06-4e7e-9a4a-6c954422b5b2\"}],\"packageUris\":[\"http://schema.mathworks.com/mf0/Connector/R2020b\"],\"version\":\"1.0\"}"
  Limb_Segment2 : Subsystem
      settings: PortSchema="{\"entries\":[{\"content\":{\"sides\":[{\"content\":{\"connectorIds\":[\"In1\",\"In2\",\"In3\",\"In4\"]},\"type\":\"ConnectorPlacement.EquallySpacedRectSide\",\"uuid\":\"d6f10fa6-a397-4eb1-90c1-ee7478ada294\"},{\"content\":{\"side\":\"RIGHT\"},\"type\":\"ConnectorPlacement.EquallySpacedRectSide\",\"uuid\":\"3f1db35a-8e6d-4ba3-9e2d-f9910440e53b\"},{\"content\":{\"connectorIds\":[\"LConn1\"],\"side\":\"TOP\"},\"type\":\"ConnectorPlacement.EquallySpacedRectSide\",\"uuid\":\"a4104d1f-7883-4f84-b664-87694b536b33\"},{\"content\":{\"connectorIds\":[\"RConn1\"],\"side\":\"BOTTOM\"},\"type\":\"ConnectorPlacement.EquallySpacedRectSide\",\"uuid\":\"6469b369-5782-4c2c-b5b8-85624622bc1d\"}]},\"type\":\"ConnectorPlacement.EquallySpacedConnector\",\"uuid\":\"3cfa1fa9-4e06-4e7e-9a4a-6c954422b5b2\"}],\"packageUris\":[\"http://schema.mathworks.com/mf0/Connector/R2020b\"],\"version\":\"1.0\"}"
  Limb_Segment3 : Subsystem
      settings: PortSchema="{\"entries\":[{\"content\":{\"sides\":[{\"content\":{\"connectorIds\":[\"In1\",\"In2\",\"In3\",\"In4\"]},\"type\":\"ConnectorPlacement.EquallySpacedRectSide\",\"uuid\":\"d6f10fa6-a397-4eb1-90c1-ee7478ada294\"},{\"content\":{\"side\":\"RIGHT\"},\"type\":\"ConnectorPlacement.EquallySpacedRectSide\",\"uuid\":\"3f1db35a-8e6d-4ba3-9e2d-f9910440e53b\"},{\"content\":{\"connectorIds\":[\"LConn1\"],\"side\":\"TOP\"},\"type\":\"ConnectorPlacement.EquallySpacedRectSide\",\"uuid\":\"a4104d1f-7883-4f84-b664-87694b536b33\"},{\"content\":{\"connectorIds\":[\"RConn1\"],\"side\":\"BOTTOM\"},\"type\":\"ConnectorPlacement.EquallySpacedRectSide\",\"uuid\":\"6469b369-5782-4c2c-b5b8-85624622bc1d\"}]},\"type\":\"ConnectorPlacement.EquallySpacedConnector\",\"uuid\":\"3cfa1fa9-4e06-4e7e-9a4a-6c954422b5b2\"}],\"packageUris\":[\"http://schema.mathworks.com/mf0/Connector/R2020b\"],\"version\":\"1.0\"}"
  Limb_Segment4 : Subsystem
      settings: PortSchema="{\"entries\":[{\"content\":{\"sides\":[{\"content\":{\"connectorIds\":[\"In1\",\"In2\",\"In3\",\"In4\"]},\"type\":\"ConnectorPlacement.EquallySpacedRectSide\",\"uuid\":\"d6f10fa6-a397-4eb1-90c1-ee7478ada294\"},{\"content\":{\"side\":\"RIGHT\"},\"type\":\"ConnectorPlacement.EquallySpacedRectSide\",\"uuid\":\"3f1db35a-8e6d-4ba3-9e2d-f9910440e53b\"},{\"content\":{\"connectorIds\":[\"LConn1\"],\"side\":\"TOP\"},\"type\":\"ConnectorPlacement.EquallySpacedRectSide\",\"uuid\":\"a4104d1f-7883-4f84-b664-87694b536b33\"},{\"content\":{\"connectorIds\":[\"RConn1\"],\"side\":\"BOTTOM\"},\"type\":\"ConnectorPlacement.EquallySpacedRectSide\",\"uuid\":\"6469b369-5782-4c2c-b5b8-85624622bc1d\"}]},\"type\":\"ConnectorPlacement.EquallySpacedConnector\",\"uuid\":\"3cfa1fa9-4e06-4e7e-9a4a-6c954422b5b2\"}],\"packageUris\":[\"http://schema.mathworks.com/mf0/Connector/R2020b\"],\"version\":\"1.0\"}"
  Limb_Segment5 : Subsystem
      settings: PortSchema="{\"entries\":[{\"content\":{\"sides\":[{\"content\":{\"connectorIds\":[\"In1\",\"In2\",\"In3\",\"In4\"]},\"type\":\"ConnectorPlacement.EquallySpacedRectSide\",\"uuid\":\"d6f10fa6-a397-4eb1-90c1-ee7478ada294\"},{\"content\":{\"side\":\"RIGHT\"},\"type\":\"ConnectorPlacement.EquallySpacedRectSide\",\"uuid\":\"3f1db35a-8e6d-4ba3-9e2d-f9910440e53b\"},{\"content\":{\"connectorIds\":[\"LConn1\"],\"side\":\"TOP\"},\"type\":\"ConnectorPlacement.EquallySpacedRectSide\",\"uuid\":\"a4104d1f-7883-4f84-b664-87694b536b33\"},{\"content\":{\"connectorIds\":[\"RConn1\"],\"side\":\"BOTTOM\"},\"type\":\"ConnectorPlacement.EquallySpacedRectSide\",\"uuid\":\"6469b369-5782-4c2c-b5b8-85624622bc1d\"}]},\"type\":\"ConnectorPlacement.EquallySpacedConnector\",\"uuid\":\"3cfa1fa9-4e06-4e7e-9a4a-6c954422b5b2\"}],\"packageUris\":[\"http://schema.mathworks.com/mf0/Connector/R2020b\"],\"version\":\"1.0\"}"
  Limb_Segment6 : Subsystem
      settings: PortSchema="{\"entries\":[{\"content\":{\"sides\":[{\"content\":{\"connectorIds\":[\"In1\",\"In2\",\"In3\",\"In4\"]},\"type\":\"ConnectorPlacement.EquallySpacedRectSide\",\"uuid\":\"d6f10fa6-a397-4eb1-90c1-ee7478ada294\"},{\"content\":{\"side\":\"RIGHT\"},\"type\":\"ConnectorPlacement.EquallySpacedRectSide\",\"uuid\":\"3f1db35a-8e6d-4ba3-9e2d-f9910440e53b\"},{\"content\":{\"connectorIds\":[\"LConn1\"],\"side\":\"TOP\"},\"type\":\"ConnectorPlacement.EquallySpacedRectSide\",\"uuid\":\"a4104d1f-7883-4f84-b664-87694b536b33\"},{\"content\":{\"connectorIds\":[\"RConn1\"],\"side\":\"BOTTOM\"},\"type\":\"ConnectorPlacement.EquallySpacedRectSide\",\"uuid\":\"6469b369-5782-4c2c-b5b8-85624622bc1d\"}]},\"type\":\"ConnectorPlacement.EquallySpacedConnector\",\"uuid\":\"3cfa1fa9-4e06-4e7e-9a4a-6c954422b5b2\"}],\"packageUris\":[\"http://schema.mathworks.com/mf0/Connector/R2020b\"],\"version\":\"1.0\"}"
  Limb_Segment7 : Subsystem
      settings: PortSchema="{\"entries\":[{\"content\":{\"sides\":[{\"content\":{\"connectorIds\":[\"In1\",\"In2\",\"In3\",\"In4\"]},\"type\":\"ConnectorPlacement.EquallySpacedRectSide\",\"uuid\":\"d6f10fa6-a397-4eb1-90c1-ee7478ada294\"},{\"content\":{\"side\":\"RIGHT\"},\"type\":\"ConnectorPlacement.EquallySpacedRectSide\",\"uuid\":\"3f1db35a-8e6d-4ba3-9e2d-f9910440e53b\"},{\"content\":{\"connectorIds\":[\"LConn1\"],\"side\":\"TOP\"},\"type\":\"ConnectorPlacement.EquallySpacedRectSide\",\"uuid\":\"a4104d1f-7883-4f84-b664-87694b536b33\"},{\"content\":{\"connectorIds\":[\"RConn1\"],\"side\":\"BOTTOM\"},\"type\":\"ConnectorPlacement.EquallySpacedRectSide\",\"uuid\":\"6469b369-5782-4c2c-b5b8-85624622bc1d\"}]},\"type\":\"ConnectorPlacement.EquallySpacedConnector\",\"uuid\":\"3cfa1fa9-4e06-4e7e-9a4a-6c954422b5b2\"}],\"packageUris\":[\"http://schema.mathworks.com/mf0/Connector/R2020b\"],\"version\":\"1.0\"}"
  Limb_Segment8 : Subsystem
      settings: PortSchema="{\"entries\":[{\"content\":{\"sides\":[{\"content\":{\"connectorIds\":[\"In1\",\"In2\",\"In3\",\"In4\"]},\"type\":\"ConnectorPlacement.EquallySpacedRectSide\",\"uuid\":\"d6f10fa6-a397-4eb1-90c1-ee7478ada294\"},{\"content\":{\"side\":\"RIGHT\"},\"type\":\"ConnectorPlacement.EquallySpacedRectSide\",\"uuid\":\"3f1db35a-8e6d-4ba3-9e2d-f9910440e53b\"},{\"content\":{\"connectorIds\":[\"LConn1\"],\"side\":\"TOP\"},\"type\":\"ConnectorPlacement.EquallySpacedRectSide\",\"uuid\":\"a4104d1f-7883-4f84-b664-87694b536b33\"},{\"content\":{\"connectorIds\":[\"RConn1\"],\"side\":\"BOTTOM\"},\"type\":\"ConnectorPlacement.EquallySpacedRectSide\",\"uuid\":\"6469b369-5782-4c2c-b5b8-85624622bc1d\"}]},\"type\":\"ConnectorPlacement.EquallySpacedConnector\",\"uuid\":\"3cfa1fa9-4e06-4e7e-9a4a-6c954422b5b2\"}],\"packageUris\":[\"http://schema.mathworks.com/mf0/Connector/R2020b\"],\"version\":\"1.0\"}"
  Limb_Segment9 : Subsystem
      settings: PortSchema="{\"entries\":[{\"content\":{\"sides\":[{\"content\":{\"connectorIds\":[\"In1\",\"In2\",\"In3\",\"In4\"]},\"type\":\"ConnectorPlacement.EquallySpacedRectSide\",\"uuid\":\"d6f10fa6-a397-4eb1-90c1-ee7478ada294\"},{\"content\":{\"side\":\"RIGHT\"},\"type\":\"ConnectorPlacement.EquallySpacedRectSide\",\"uuid\":\"3f1db35a-8e6d-4ba3-9e2d-f9910440e53b\"},{\"content\":{\"connectorIds\":[\"LConn1\"],\"side\":\"TOP\"},\"type\":\"ConnectorPlacement.EquallySpacedRectSide\",\"uuid\":\"a4104d1f-7883-4f84-b664-87694b536b33\"},{\"content\":{\"connectorIds\":[\"RConn1\"],\"side\":\"BOTTOM\"},\"type\":\"ConnectorPlacement.EquallySpacedRectSide\",\"uuid\":\"6469b369-5782-4c2c-b5b8-85624622bc1d\"}]},\"type\":\"ConnectorPlacement.EquallySpacedConnector\",\"uuid\":\"3cfa1fa9-4e06-4e7e-9a4a-6c954422b5b2\"}],\"packageUris\":[\"http://schema.mathworks.com/mf0/Connector/R2020b\"],\"version\":\"1.0\"}"
  MATLAB Function2 : MATLAB Function  TreatAsAtomicUnit=on
  PS-Simulink Converter : nesl_utility/PS-Simulink Converter  PhysicalDomain=network_engine_domain  SubClassName=ps_output  LeftPortType=input  RightPortType=output  PseudoPeriodic=off  Frequencies=[]  VectorFormat=inherit  Unit=inherit  AffineConversion=off
  Product{,1..3} (4 alike) : Product
  Right Ball Contact : Subsystem
  SMA1 F(V) : Subsystem
  SMA2 F(V) : Subsystem
  SMA3 F(V) : Subsystem
  SMA4 F(V) : Subsystem
  Terminator : Terminator
  Transform Sensor : sm_lib/Frames and Transforms/Transform Sensor  MeasurementFrame=Base  RotationSequence=XYZ  SenseAngle=off  SenseAxis=off  SenseQ=off  SenseR=on  SenseRotationSequence=off  SenseOmegaX=off  SenseOmegaY=off  SenseOmegaZ=off  SenseOmega=off  SenseQDot=off  SenseRDot=off  SenseRotationSequenceDot=off  SenseAlphaX=off  SenseAlphaY=off  SenseAlphaZ=off  SenseAlpha=off  SenseQDDot=off  SenseRDDot=off  SenseX=off  SenseY=off  SenseZ=off  SenseXYZ=off  SenseRad=off  SenseAzim=off  SenseDist=off  SenseInc=off  SenseXDot=off  SenseYDot=off  SenseZDot=off  SenseXYZDot=off  SenseRadDot=off  SenseAzimDot=off  SenseDistDot=off  SenseIncDot=off  SenseXDDot=off  SenseYDDot=off  SenseZDDot=off  SenseXYZDDot=off  SenseRadDDot=off  SenseAzimDDot=off  SenseDistDDot=off  SenseIncDDot=off
  Base1 : PMIOPort  Side=Left
  theta_X : Outport
  theta_Y : Outport  Port=2
  "Contact " : Outport  Port=3
  GRF : Outport  Port=4
  GRFt : Outport  Port=5
  GRFn : Outport  Port=6
  wires:
  [F_SMA2] -> Limb_Segment4/2(In2)
  [F_SMA2] -> Limb_Segment3/2(In2)
  [F_SMA1] -> Limb_Segment1/1(In1)
  [F_SMA2] -> Limb_Segment8/2(In2)
  [F_SMA3] -> Limb_Segment2/3(In3)
  SMA3 F(V)/1(F) -> [F_SMA3]
  [F_SMA3] -> Limb_Segment1/3(In3)
  [F_SMA2] -> Limb_Segment9/2(In2)
  Constant2/1 -> Product2/2
  [F_SMA1] -> Limb_Segment6/1(In1)
  SMA1 F(V)/1(F) -> [F_SMA1]
  [F_SMA4] -> Limb_Segment8/4(In4)
  [F_SMA3] -> Limb_Segment5/3(In3)
  [F_SMA3] -> Limb_Segment7/3(In3)
  Constant/1 -> Product/2
  [F_SMA4] -> Limb_Segment4/4(In4)
  [F_SMA4] -> Limb_Segment5/4(In4)
  [F_SMA4] -> Limb_Segment1/4(In4)
  [F_SMA4] -> Limb_Segment3/4(In4)
  [F_SMA3] -> Limb_Segment/3(In3)
  [F_SMA2] -> Limb_Segment/2(In2)
  [F_SMA3] -> Limb_Segment4/3(In3)
  [F_SMA1] -> Limb_Segment2/1(In1)
  [F_SMA2] -> Limb_Segment1/2(In2)
  [F_SMA3] -> Limb_Segment9/3(In3)
  Product2/1 -> SMA3 F(V)/1(V_1)  "Input Voltage 3"
  SMA2 F(V)/1(F) -> [F_SMA2]
  [F_SMA2] -> Limb_Segment2/2(In2)
  [F_SMA2] -> Limb_Segment7/2(In2)
  [F_SMA1] -> Limb_Segment4/1(In1)
  [F_SMA1] -> Limb_Segment5/1(In1)
  Duty Cycle 4/1 -> Product3/1
  [F_SMA1] -> Limb_Segment3/1(In1)
  [F_SMA1] -> Limb_Segment8/1(In1)
  [F_SMA3] -> Limb_Segment8/3(In3)
  [F_SMA4] -> Limb_Segment6/4(In4)
  PS-Simulink Converter/1 -> MATLAB Function2/1(R)
  [F_SMA1] -> Limb_Segment/1(In1)
  Product3/1 -> SMA4 F(V)/1(V_1)  "Input Voltage 4"
  [F_SMA2] -> Limb_Segment6/2(In2)
  [F_SMA3] -> Limb_Segment3/3(In3)
  Constant1/1 -> Product1/2
  [F_SMA4] -> Limb_Segment9/4(In4)
  [F_SMA1] -> Limb_Segment9/1(In1)
  SMA4 F(V)/1(F) -> [F_SMA4]
  [F_SMA3] -> Limb_Segment6/3(In3)
  [F_SMA1] -> Limb_Segment7/1(In1)
  [F_SMA4] -> Limb_Segment2/4(In4)
  [F_SMA4] -> Limb_Segment/4(In4)
  [F_SMA4] -> Limb_Segment7/4(In4)
  [F_SMA2] -> Limb_Segment5/2(In2)
  Constant3/1 -> Product3/2
  Product/1 -> SMA1 F(V)/1(V_1)  "Input Voltage1"
  MATLAB Function2/3(yaw_deg) -> Terminator/1  "theta_Z"
  Product1/1 -> SMA2 F(V)/1(V_1)  "Input Voltage 2"
  Duty Cycle 3/1 -> Product2/1
  Duty Cycle 2/1 -> Product1/1
  MATLAB Function2/2(pitch_deg) -> theta_Y/1  "theta_Y"
  MATLAB Function2/1(roll_deg) -> theta_X/1  "theta_X"
  Duty Cycle 1/1 -> Product/1
  Right Ball Contact/2(GRF [N N N]) -> GRF/1
  Right Ball Contact/4(GRFn [N N N]) -> GRFn/1
  Right Ball Contact/1(RBallContact [bool]) -> "Contact "/1
  Right Ball Contact/3(GRFt [N N N]) -> GRFt/1
  connections:
  Transform Sensor/LConn1 -- Base1/RConn1 -- Base/RConn1 -- Limb_Segment/LConn1
  Limb_Segment2/LConn1 -- Limb_Segment1/RConn1
  Limb_Segment8/RConn1 -- Limb_Segment9/LConn1
  Limb_Segment3/LConn1 -- Limb_Segment2/RConn1
  Limb_Segment4/LConn1 -- Limb_Segment3/RConn1
  Limb_Segment6/LConn1 -- Limb_Segment5/RConn1
  Limb_Segment8/LConn1 -- Limb_Segment7/RConn1
  Transform Sensor/RConn1 -- Right Ball Contact/LConn1 -- Limb_Segment9/RConn1
  Limb_Segment7/LConn1 -- Limb_Segment6/RConn1
  Limb_Segment4/RConn1 -- Limb_Segment5/LConn1
  Limb_Segment1/LConn1 -- Limb_Segment/RConn1
  PS-Simulink Converter/LConn1 -- Transform Sensor/RConn2
